simulink model "ayonlab6"  (R2020a)
settings: Solver=VariableStepAuto  StartTime=0.0  StopTime=10.0  RelTol=1e-3  EnableMultiTasking=on
settings Model: Creator=Student  LastModifiedBy=hp
settings DataIOCC: ReturnWorkspaceOutputs=off
settings OptimizationCC: LifeSpan=inf
settings DebuggingCC: SFUnexpectedBacktrackingDiag=warning  SFNoUnconditionalDefaultTransitionDiag=warning  ArithmeticOperatorsInVariantConditions=warning
settings SFSimCC: SimUseLocalCustomCode=off  CustomCodeUndefinedFunction=UseInterfaceOnly
settings RTWCC: RTWUseLocalCustomCode=off
settings CodeAppCC: StateflowObjectComments=on
settings GRTTargetCC: TargetLangStandard=C89/C90 (ANSI)
settings ConfigComp: CovMetricSettings=dw  CovHtmlReporting=on  CovSaveCumulativeToWorkspaceVar=on  CovSaveSingleToWorkspaceVar=on  CovExternalEMLEnable=off

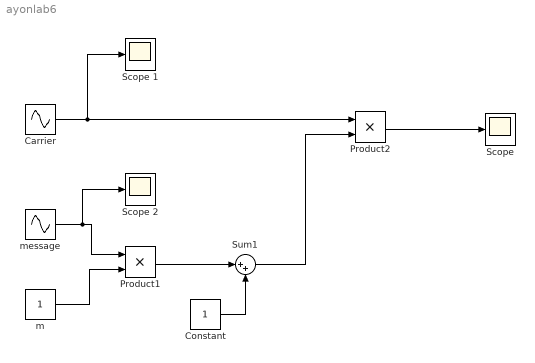
== system ayonlab6 ==
  Carrier : Sin  Amplitude=5  Frequency=2*pi*25  SampleTime=1/5000
  Constant : Constant
  "Product1 " : Product
  Product2 : Product
  "Scope " : Scope
  Scope 1 : Scope
  Scope 2 : Scope
  Sum1 : Sum  Inputs=|++
  m : Constant
  message : Sin  Frequency=2*pi  SampleTime=1/5000
  wires:
  message/1 -> Scope 2/1, "Product1 "/1
  m/1 -> "Product1 "/2
  Carrier/1 -> Scope 1/1, Product2/1
  "Product1 "/1 -> Sum1/1
  Constant/1 -> Sum1/2
  Sum1/1 -> Product2/2
  Product2/1 -> "Scope "/1
